simulink model "Problem_16_6"  (Simulink 7.5)
settings: Solver=ode45  StartTime=0.0  StopTime=10.0  RelTol=1e-3
settings Model: Creator=Holly  LastModifiedBy=Holly

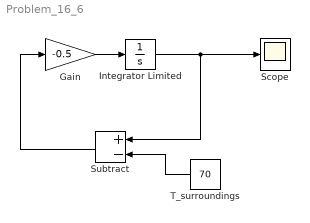
== system Problem_16_6 ==
  Gain : Gain  Gain=-0.5  ParameterDataType=fixdt(1, 16)  ParameterScaling=2^0  OutDataType=fixdt(1, 16)  OutScaling=2^0
  Integrator Limited : Integrator  InitialCondition=110  UpperSaturationLimit=1  LowerSaturationLimit=0
  Scope : Scope
  Subtract : Sum  Inputs=+-  OutDataType=fixdt(1, 16)  OutScaling=2^-10
  T_surroundings : Constant  Value=70  OutDataType=fixdt(1, 16)  OutScaling=2^0
  wires:
  Integrator Limited/1 -> Scope/1, Subtract/1
  T_surroundings/1 -> Subtract/2
  Gain/1 -> Integrator Limited/1
  Subtract/1 -> Gain/1
